simulink model "Teste_ModeloPV_2015a"  (R2015a)
settings: Solver=ode45  SolverMode=SingleTasking  StartTime=0.0  StopTime=100  MaxStep=1e-2  MinStep=1e-8  RelTol=1e-3
libraries: simulink x3, AvgModels x1
settings Model: CovMetricSettings=dwe  CovHtmlReporting=off  covSaveCumulativeToWorkspaceVar=off  CovSaveSingleToWorkspaceVar=off  CovExternalEMLEnable=on  Creator=lgalotto  LastModifiedBy=lgalo
settings DataIOCC: LimitDataPoints=off  SaveFormat=Dataset
settings DebuggingCC: SFUnexpectedBacktrackingDiag=error  SFNoUnconditionalDefaultTransitionDiag=error
settings HardwareCC: ProdBitPerPointer=64  ProdLargestAtomicFloat=Float  ProdIntDivRoundTo=Zero  ProdEndianess=LittleEndian  ProdHWDeviceType=Specified
settings ModelReferenceCC: PropagateSignalLabelsOutOfModel=on
settings GRTTargetCC: TargetLangStandard=C99 (ISO)  GeneratePreprocessorConditionals=Use local settings

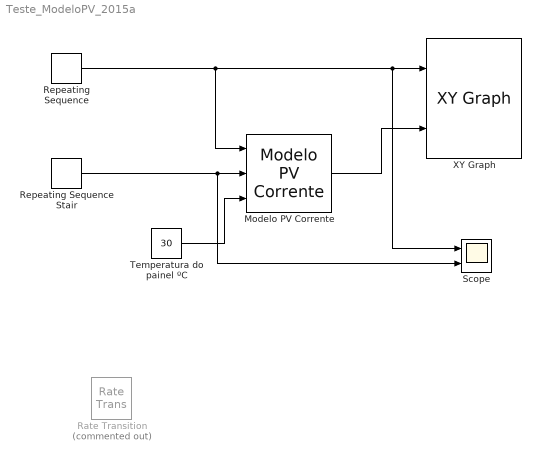
== system Teste_ModeloPV_2015a ==
  Modelo PV Corrente : AvgModels/Modelo PV Corrente  Ms=1  Mp=1  Ns=54  Voc=0.6093  Isc=8.21  Tr=273 + 25  tau=1e-3  Rs=0.005  Rp=7  a=3.18e-3  n=1.2  k=1.38e-23  q=1.60e-19  EG=1.1
  Rate Transition : RateTransition  Commented=on  OutPortSampleTime=0.001
  Repeating Sequence : simulink/Sources/Repeating Sequence  rep_seq_t=[0 5 10]  rep_seq_y=[32 0 32]
  Repeating Sequence Stair : simulink/Sources/Repeating Sequence Stair  OutValues=[100 200 300 400 500 600 700 800 900 1000].'  tsamp=10  OutMin=[]  OutMax=[]  OutDataTypeStr=double  OutputDataTypeScalingMode=double  OutDataType=fixdt(0,8)  ConRadixGroup=Best Precision: Vector-wise  OutScaling=2^-12
  Scope : Scope  NumInputPorts=2
      settings: YMin=-4.00000~-125.00000  YMax=36.00000~1125.00000
  Temperatura do painel ºC : Constant  Value=30
  XY Graph : simulink/Sinks/XY Graph  xmin=0  xmax=32  ymin=0  ymax=10  st=-1
  wires:
  Temperatura do painel ºC/1 -> Modelo PV Corrente/3
  Repeating Sequence/1 -> Modelo PV Corrente/1, Scope/1, XY Graph/1
  Modelo PV Corrente/1 -> XY Graph/2
  Repeating Sequence Stair/1 -> Scope/2, Modelo PV Corrente/2
